simulink model "test_filtro"  (R2018a)
settings: Solver=FixedStepDiscrete  StartTime=0.0  StopTime=inf  RelTol=1e-3
values from neighbouring files (symbols this model uses):
  k = 0.001    [obs_zaki.m]
undefined symbols (not defined in the file or in its folder): K
settings Model: Creator=facu  LastModifiedBy=facu
settings SolverCC: AutoInsertRateTranBlk=on
settings DataIOCC: LimitDataPoints=on  SaveOutput=off  SignalLogging=off  DSMLogging=off  SaveTime=off
settings OptimizationCC: LifeSpan=inf
settings DebuggingCC: AlgebraicLoopMsg=error  SingleTaskRateTransMsg=error  AllowSymbolicDim=off  SFUnexpectedBacktrackingDiag=warning  SFNoUnconditionalDefaultTransitionDiag=warning  SFExecutionAtInitializationDiag=none
settings CodeAppCC: StateflowObjectComments=on
settings GRTTargetCC: TargetLangStandard=C89/C90 (ANSI)  GeneratePreprocessorConditionals=Disable all

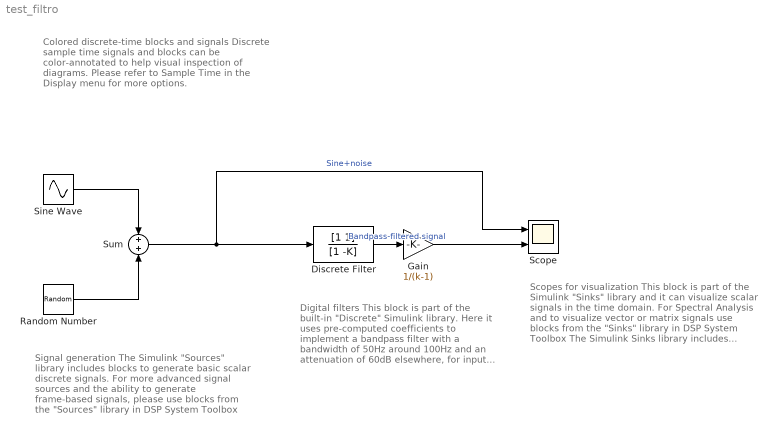
== system test_filtro ==
  note: Signal generation
      | The Simulink "Sources" library includes blocks to generate basic scalar discrete signals.
      | For more advanced signal sources and the ability to generate frame-based signals, please use blocks from the "Sources" library in DSP System Toolbox
  note: Scopes for visualization
      | This block is part of the Simulink "Sinks" library and it can visualize scalar signals in the time domain.
      | For Spectral Analysis and to visualize vector or matrix signals use blocks from the "Sinks" library in DSP System Toolbox
      |
      | The Simulink Sinks library includes scopes to visualize scalar signals in the time domain. For the Spectrum Analyzer and to viasualize vector or matrix signals refer to the Sinks library of DSP System Toolbox
  note: Digital filters
      | This block is part of the built-in "Discrete" Simulink library. Here it uses pre-computed coefficients to implement a bandpass filter with a bandwidth of 50Hz around 100Hz and an attenuation of 60dB elsewhere, for input signals sampled at 8kHz.
      | To design digital filters, to select specific implementation structures, or to simulate fixed-point arithmetic use blocks from the "Filtering" library in DSP System Toolbox
  note: Colored discrete-time blocks and signals
      | Discrete sample time signals and blocks can be color-annotated to help visual inspection of diagrams. Please refer to Sample Time in the Display menu for more options.
  Discrete Filter : DiscreteFilter  Numerator=[1 1]  Denominator=[1 -K]
  Gain : Gain  Gain=1/(k-1)
  Random Number : RandomNumber  SampleTime=1/8000
  Scope : Scope  NumInputPorts=2
  Sine Wave : Sin  Frequency=2*pi*100  Samples=1  SampleTime=1/8000
  Sum : Sum
  wires:
  Discrete Filter/1 -> Gain/1  "Bandpass-filtered signal"
  Sum/1 -> Discrete Filter/1, Scope/1  "Sine+noise"
  Sine Wave/1 -> Sum/1
  Random Number/1 -> Sum/2
  Gain/1 -> Scope/2
